simulink library "McControllerLibrary"  (R2026a)
settings: Solver=VariableStepAuto
undefined symbols (not defined in the file): McControl_Params, McRuntime_Init
settings Model: Creator=k  LastModifiedBy=k

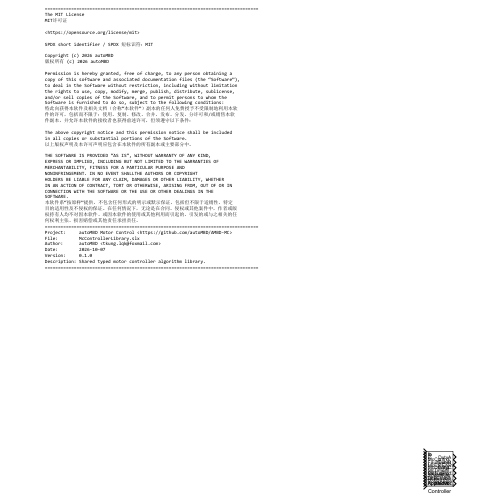
[thumbnail: Simulink's stored preview of the top-level diagram]
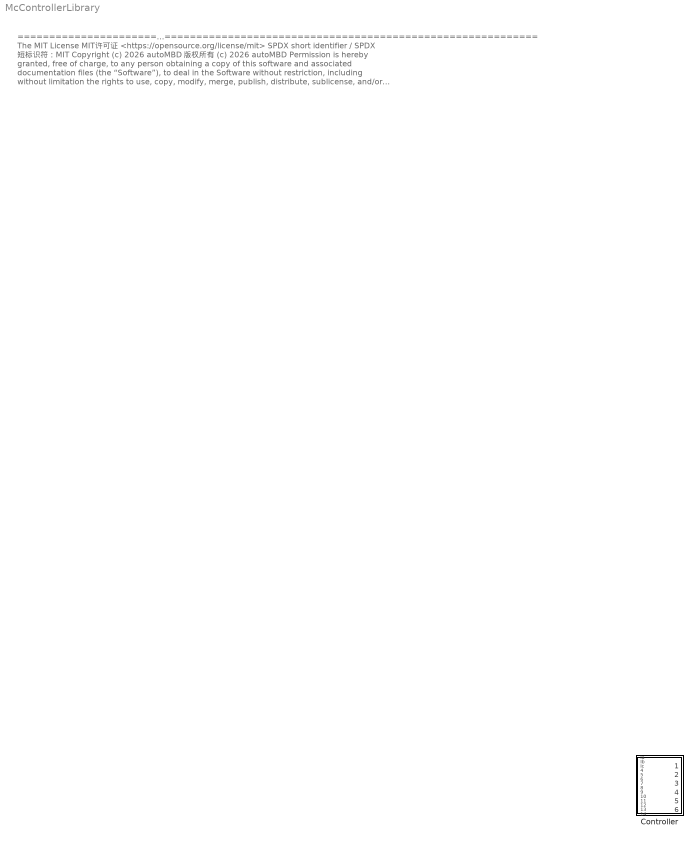
== system McControllerLibrary ==
  note: =================================================================================
      | The MIT License
      | MIT许可证
      |
      | <https://opensource.org/license/mit>
      |
      | SPDX short identifier / SPDX 短标识符：MIT
      |
      | Copyright (c) 2026 autoMBD
      | 版权所有 (c) 2026 autoMBD
      |
      | Permission is hereby granted, free of charge, to any person obtaining a
      | copy of this software and associated documentation files (the “Software”),
      | to deal in the Software without restriction, including without limitation
      | the rights to use, copy, modify, merge, publish, distribute, sublicense,
      | and/or sell copies of the Software, and to permit persons to whom the
      | Software is furnished to do so, subject to the following conditions:
      | 特此向获得本软件及相关文档（合称“本软件”）副本的任何人免费授予不受限制地利用本软
      | 件的许可，包括而不限于：使用、复制、修改、合并、发布、分发、分许可和/或销售本软
      | 件副本，并允许本软件的接收者也获得前述许可，但须遵守以下条件：
      |
      | The above copyright notice and this permission notice shall be included
      | in all copies or substantial portions of the Software.
      | 以上版权声明及本许可声明应包含在本软件的所有副本或主要部分中。
      |
      | THE SOFTWARE IS PROVIDED “AS IS”, WITHOUT WARRANTY OF ANY KIND,
      | EXPRESS OR IMPLIED, INCLUDING BUT NOT LIMITED TO THE WARRANTIES OF
      | MERCHANTABILITY, FITNESS FOR A PARTICULAR PURPOSE AND
      | NONINFRINGEMENT. IN NO EVENT SHALLTHE AUTHORS OR COPYRIGHT
      | HOLDERS BE LIABLE FOR ANY CLAIM, DAMAGES OR OTHER LIABILITY, WHETHER
      | IN AN ACTION OF CONTRACT, TORT OR OTHERWISE, ARISING FROM, OUT OF OR IN
      | CONNECTION WITH THE SOFTWARE OR THE USE OR OTHER DEALINGS IN THE
      | SOFTWARE.
      | 本软件系“按原样”提供，不包含任何形式的明示或默示保证，包括但不限于适销性、特定
      | 目的适用性及不侵权的保证。在任何情况下，无论是在合同、侵权或其他案件中，作者或版
      | 权持有人均不对因本软件、或因本软件的使用或其他利用而引起的、引发的或与之相关的任
      | 何权利主张、损害赔偿或其他责任承担责任。
      | =================================================================================
      | Project:     autoMBD Motor Control <https://github.com/autoMBD/AMBD-MC>
      | File:        McControllerLibrary.slx
      | Author:      autoMBD <tkung.lqk@foxmail.com>
      | Date:        2026-10-07
      | Version:     0.1.0
      | Description: Shared typed motor controller algorithm library.
      | =================================================================================
  Controller : Subsystem

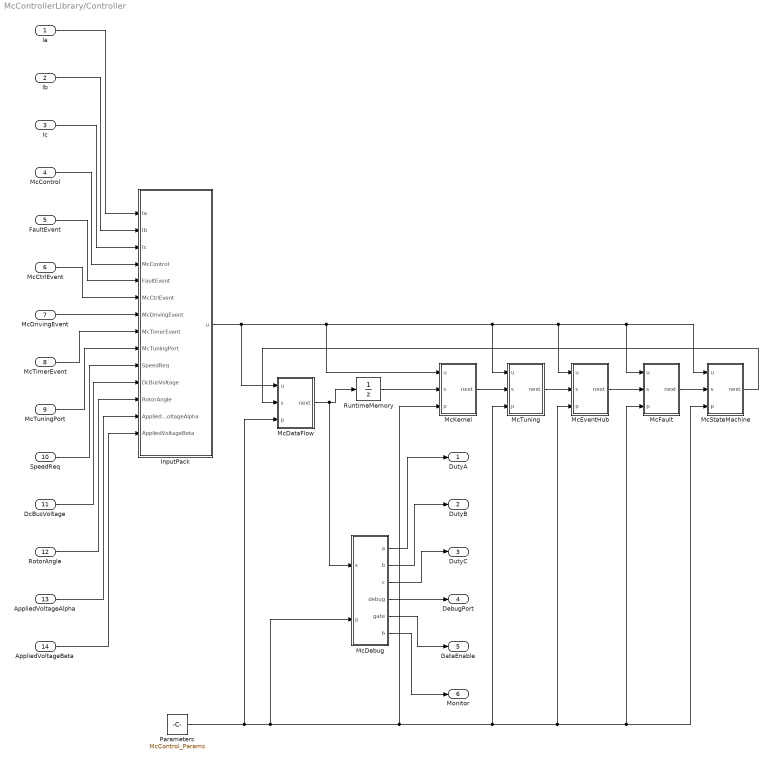
== system McControllerLibrary/Controller ==
  Ia : Inport  OutDataTypeStr=uint16  SampleTime=6.25e-5
  Ib : Inport  Port=2  OutDataTypeStr=uint16  SampleTime=6.25e-5
  Ic : Inport  Port=3  OutDataTypeStr=uint16  SampleTime=6.25e-5
  McControl : Inport  Port=4  OutDataTypeStr=uint8  SampleTime=6.25e-5
  FaultEvent : Inport  Port=5  OutDataTypeStr=boolean  SampleTime=6.25e-5
  McCtrlEvent : Inport  Port=6  OutDataTypeStr=boolean  SampleTime=6.25e-5
  McDrivingEvent : Inport  Port=7  OutDataTypeStr=boolean  SampleTime=6.25e-5
  McTimerEvent : Inport  Port=8  OutDataTypeStr=boolean  SampleTime=6.25e-5
  McTuningPort : Inport  Port=9  OutDataTypeStr=Bus: tMcTuning  SampleTime=6.25e-5
  SpeedReq : Inport  Port=10  OutDataTypeStr=single  SampleTime=6.25e-5
  DcBusVoltage : Inport  Port=11  OutDataTypeStr=single  SampleTime=6.25e-5
  RotorAngle : Inport  Port=12  OutDataTypeStr=single  SampleTime=6.25e-5
  AppliedVoltageAlpha : Inport  Port=13  OutDataTypeStr=single  SampleTime=6.25e-5
  AppliedVoltageBeta : Inport  Port=14  OutDataTypeStr=single  SampleTime=6.25e-5
  InputPack : MATLAB Function  TreatAsAtomicUnit=on
  McDataFlow : Subsystem
  McDebug : MATLAB Function  TreatAsAtomicUnit=on
  McEventHub : Subsystem
  McFault : Subsystem
  McKernel : Subsystem
  McStateMachine : Subsystem
  McTuning : Subsystem
  Parameters : Constant  Value=McControl_Params  OutDataTypeStr=Bus: tMcControlParams
  RuntimeMemory : UnitDelay  InitialCondition=McRuntime_Init  SampleTime=6.25e-5
  DutyA : Outport  OutDataTypeStr=uint16
  DutyB : Outport  Port=2  OutDataTypeStr=uint16
  DutyC : Outport  Port=3  OutDataTypeStr=uint16
  DebugPort : Outport  Port=4  OutDataTypeStr=Bus: tMcDebug
  GateEnable : Outport  Port=5  OutDataTypeStr=boolean
  Monitor : Outport  Port=6  OutDataTypeStr=Bus: tMcMonitor
  wires:
  McDebug/6(monitor) -> Monitor/1
  McDebug/5(gate) -> GateEnable/1
  McDebug/4(debug) -> DebugPort/1
  McDebug/3(c) -> DutyC/1
  McDebug/2(b) -> DutyB/1
  McDebug/1(a) -> DutyA/1
  McDataFlow/1(next) -> McDebug/1(s), RuntimeMemory/1
  McStateMachine/1(next) -> McDataFlow/2(s)
  McFault/1(next) -> McStateMachine/2(s)
  McEventHub/1(next) -> McFault/2(s)
  McTuning/1(next) -> McEventHub/2(s)
  McKernel/1(next) -> McTuning/2(s)
  Parameters/1 -> McStateMachine/3(p), McFault/3(p), McEventHub/3(p), McTuning/3(p), McKernel/3(p), McDebug/2(p), McDataFlow/3(p)
  RuntimeMemory/1 -> McKernel/2(s)
  InputPack/1(u) -> McFault/1(u), McStateMachine/1(u), McEventHub/1(u), McTuning/1(u), McKernel/1(u), McDataFlow/1(u)
  AppliedVoltageBeta/1 -> InputPack/14(AppliedVoltageBeta)
  AppliedVoltageAlpha/1 -> InputPack/13(AppliedVoltageAlpha)
  RotorAngle/1 -> InputPack/12(RotorAngle)
  DcBusVoltage/1 -> InputPack/11(DcBusVoltage)
  SpeedReq/1 -> InputPack/10(SpeedReq)
  McTuningPort/1 -> InputPack/9(McTuningPort)
  McTimerEvent/1 -> InputPack/8(McTimerEvent)
  McDrivingEvent/1 -> InputPack/7(McDrivingEvent)
  McCtrlEvent/1 -> InputPack/6(McCtrlEvent)
  FaultEvent/1 -> InputPack/5(FaultEvent)
  McControl/1 -> InputPack/4(McControl)
  Ic/1 -> InputPack/3(Ic)
  Ib/1 -> InputPack/2(Ib)
  Ia/1 -> InputPack/1(Ia)

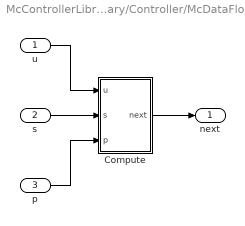
== system McControllerLibrary/Controller/McDataFlow ==
  u : Inport  OutDataTypeStr=Bus: tMcInput  SampleTime=6.25e-5
  s : Inport  Port=2  OutDataTypeStr=Bus: tMcRuntime  SampleTime=6.25e-5
  p : Inport  Port=3  OutDataTypeStr=Bus: tMcControlParams  SampleTime=6.25e-5
  Compute : MATLAB Function  TreatAsAtomicUnit=on
  next : Outport  OutDataTypeStr=Bus: tMcRuntime
  wires:
  Compute/1(next) -> next/1
  p/1 -> Compute/3(p)
  s/1 -> Compute/2(s)
  u/1 -> Compute/1(u)

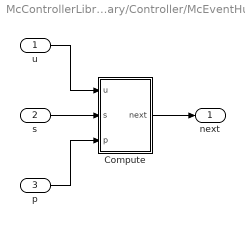
== system McControllerLibrary/Controller/McEventHub ==
  u : Inport  OutDataTypeStr=Bus: tMcInput  SampleTime=6.25e-5
  s : Inport  Port=2  OutDataTypeStr=Bus: tMcRuntime  SampleTime=6.25e-5
  p : Inport  Port=3  OutDataTypeStr=Bus: tMcControlParams  SampleTime=6.25e-5
  Compute : MATLAB Function  TreatAsAtomicUnit=on
  next : Outport  OutDataTypeStr=Bus: tMcRuntime
  wires:
  Compute/1(next) -> next/1
  p/1 -> Compute/3(p)
  s/1 -> Compute/2(s)
  u/1 -> Compute/1(u)

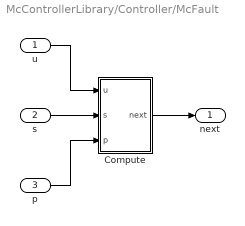
== system McControllerLibrary/Controller/McFault ==
  u : Inport  OutDataTypeStr=Bus: tMcInput  SampleTime=6.25e-5
  s : Inport  Port=2  OutDataTypeStr=Bus: tMcRuntime  SampleTime=6.25e-5
  p : Inport  Port=3  OutDataTypeStr=Bus: tMcControlParams  SampleTime=6.25e-5
  Compute : MATLAB Function  TreatAsAtomicUnit=on
  next : Outport  OutDataTypeStr=Bus: tMcRuntime
  wires:
  Compute/1(next) -> next/1
  p/1 -> Compute/3(p)
  s/1 -> Compute/2(s)
  u/1 -> Compute/1(u)

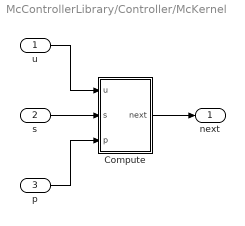
== system McControllerLibrary/Controller/McKernel ==
  u : Inport  OutDataTypeStr=Bus: tMcInput  SampleTime=6.25e-5
  s : Inport  Port=2  OutDataTypeStr=Bus: tMcRuntime  SampleTime=6.25e-5
  p : Inport  Port=3  OutDataTypeStr=Bus: tMcControlParams  SampleTime=6.25e-5
  Compute : MATLAB Function  TreatAsAtomicUnit=on
  next : Outport  OutDataTypeStr=Bus: tMcRuntime
  wires:
  Compute/1(next) -> next/1
  p/1 -> Compute/3(p)
  s/1 -> Compute/2(s)
  u/1 -> Compute/1(u)

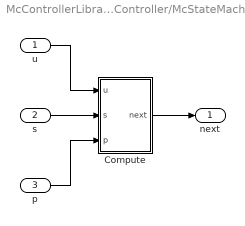
== system McControllerLibrary/Controller/McStateMachine ==
  u : Inport  OutDataTypeStr=Bus: tMcInput  SampleTime=6.25e-5
  s : Inport  Port=2  OutDataTypeStr=Bus: tMcRuntime  SampleTime=6.25e-5
  p : Inport  Port=3  OutDataTypeStr=Bus: tMcControlParams  SampleTime=6.25e-5
  Compute : MATLAB Function  TreatAsAtomicUnit=on
  next : Outport  OutDataTypeStr=Bus: tMcRuntime
  wires:
  Compute/1(next) -> next/1
  p/1 -> Compute/3(p)
  s/1 -> Compute/2(s)
  u/1 -> Compute/1(u)

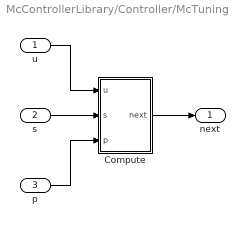
== system McControllerLibrary/Controller/McTuning ==
  u : Inport  OutDataTypeStr=Bus: tMcInput  SampleTime=6.25e-5
  s : Inport  Port=2  OutDataTypeStr=Bus: tMcRuntime  SampleTime=6.25e-5
  p : Inport  Port=3  OutDataTypeStr=Bus: tMcControlParams  SampleTime=6.25e-5
  Compute : MATLAB Function  TreatAsAtomicUnit=on
  next : Outport  OutDataTypeStr=Bus: tMcRuntime
  wires:
  Compute/1(next) -> next/1
  p/1 -> Compute/3(p)
  s/1 -> Compute/2(s)
  u/1 -> Compute/1(u)

== matlab function McControllerLibrary/Controller/McDebug ==
  data: s input; a output; p input; b output; c output; debug output Bus: tMcDebug; gate output; monitor output Bus: tMcMonitor
function [a,b,c,debug,gate,monitor]=fcn(s,p)
%#codegen
[counts,debug,monitor]=mc.monitor(s,p);
a=counts(1);b=counts(2);c=counts(3);gate=s.GateEnable;
end

== matlab function McControllerLibrary/Controller/InputPack ==
  data: Ia input; u output Bus: tMcInput; Ib input; Ic input; McControl input; FaultEvent input; McCtrlEvent input; McDrivingEvent input; McTimerEvent input; McTuningPort input; SpeedReq input; DcBusVoltage input; RotorAngle input; AppliedVoltageAlpha input; AppliedVoltageBeta input
function u=fcn(Ia,Ib,Ic,McControl,FaultEvent,McCtrlEvent,McDrivingEvent,McTimerEvent,McTuningPort,SpeedReq,DcBusVoltage,RotorAngle,AppliedVoltageAlpha,AppliedVoltageBeta)
%#codegen
u.CurrentRaw=[Ia;Ib;Ic];
u.Control=McControl;
u.Fault=FaultEvent;
u.CommandEvent=McCtrlEvent;
u.DrivingEvent=McDrivingEvent;
u.TimerEvent=McTimerEvent;
u.SpeedReq=SpeedReq;
u.Vdc=DcBusVoltage;
u.Position=RotorAngle;
u.AppliedVoltage=[AppliedVoltageAlpha;AppliedVoltageBeta];
u.Tuning=McTuningPort;
end

== matlab function McControllerLibrary/Controller/McKernel/Compute ==
  data: u input; next output Bus: tMcRuntime; s input; p input
function next=fcn(u,s,p)
%#codegen
next=mc.kernel(u,s,p);
end

== matlab function McControllerLibrary/Controller/McTuning/Compute ==
  data: u input; next output Bus: tMcRuntime; s input; p input
function next=fcn(u,s,p)
%#codegen
next=mc.tuning(u,s,p);
end

== matlab function McControllerLibrary/Controller/McEventHub/Compute ==
  data: u input; next output Bus: tMcRuntime; s input; p input
function next=fcn(u,s,p)
%#codegen
next=mc.event_hub(u,s,p);
end

== matlab function McControllerLibrary/Controller/McFault/Compute ==
  data: u input; next output Bus: tMcRuntime; s input; p input
function next=fcn(u,s,p)
%#codegen
next=mc.protection(u,s,p);
end

== matlab function McControllerLibrary/Controller/McStateMachine/Compute ==
  data: u input; next output Bus: tMcRuntime; s input; p input
function next=fcn(u,s,p)
%#codegen
next=mc.supervisor(u,s,p);
end

== matlab function McControllerLibrary/Controller/McDataFlow/Compute ==
  data: u input; next output Bus: tMcRuntime; s input; p input
function next=fcn(u,s,p)
%#codegen
next=mc.dataflow(u,s,p);
end
